simulink model "falseValue1"  (R2023a)
settings: Solver=VariableStepAuto  StartTime=0.0  StopTime=10.0  RelTol=1e-3
settings Model: Creator=Martin  LastModifiedBy=Martin

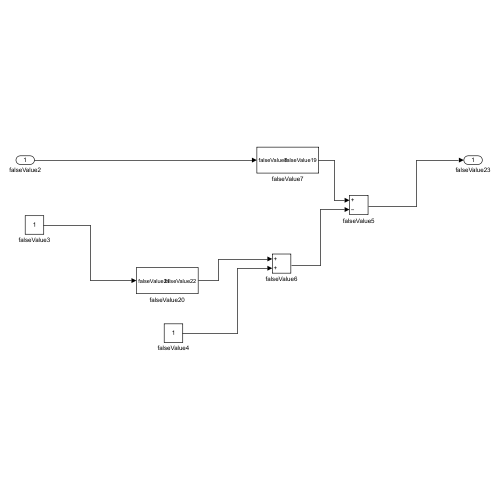
[thumbnail: Simulink's stored preview of the top-level diagram]
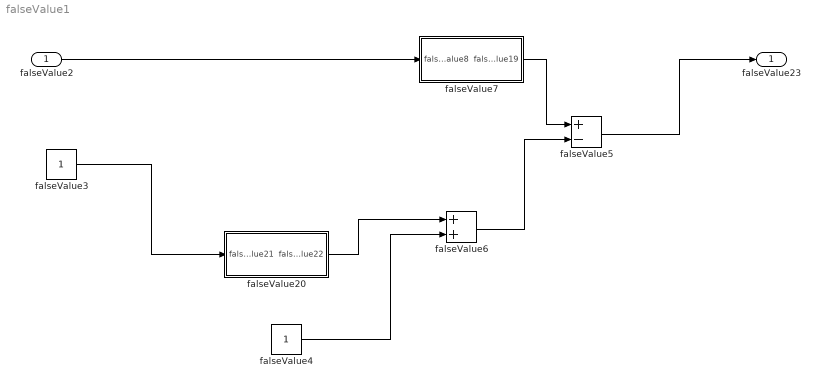
== system falseValue1 ==
  falseValue2 : Inport
  falseValue20 : Subsystem
  falseValue3 : Constant
  falseValue4 : Constant
  falseValue5 : Sum  Inputs=+-
  falseValue6 : Sum
  falseValue7 : Subsystem
  falseValue23 : Outport
  wires:
  falseValue2/1 -> falseValue7/1(falseValue8)
  falseValue5/1 -> falseValue23/1
  falseValue20/1(falseValue22) -> falseValue6/1
  falseValue4/1 -> falseValue6/2
  falseValue7/1(falseValue19) -> falseValue5/1
  falseValue6/1 -> falseValue5/2
  falseValue3/1 -> falseValue20/1(falseValue21)

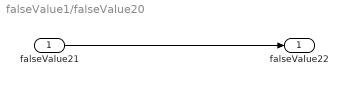
== system falseValue1/falseValue20 ==
  falseValue21 : Inport
  falseValue22 : Outport
  wires:
  falseValue21/1 -> falseValue22/1

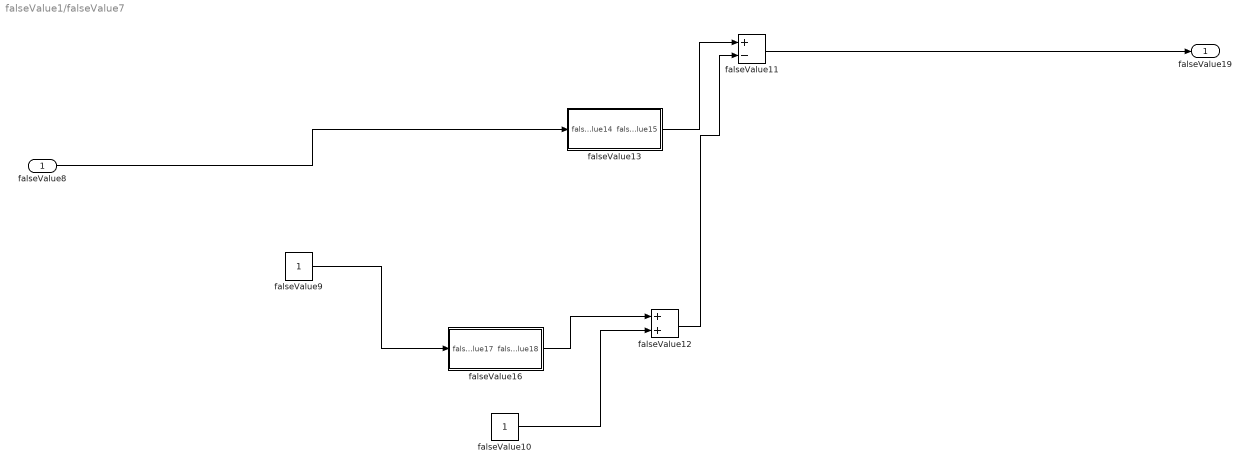
== system falseValue1/falseValue7 ==
  falseValue8 : Inport
  falseValue10 : Constant
  falseValue11 : Sum  Inputs=+-
  falseValue12 : Sum
  falseValue13 : Subsystem
  falseValue16 : Subsystem
  falseValue9 : Constant
  falseValue19 : Outport
  wires:
  falseValue9/1 -> falseValue16/1(falseValue17)
  falseValue12/1 -> falseValue11/2
  falseValue10/1 -> falseValue12/2
  falseValue16/1(falseValue18) -> falseValue12/1
  falseValue13/1(falseValue15) -> falseValue11/1
  falseValue8/1 -> falseValue13/1(falseValue14)
  falseValue11/1 -> falseValue19/1

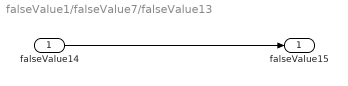
== system falseValue1/falseValue7/falseValue13 ==
  falseValue14 : Inport
  falseValue15 : Outport
  wires:
  falseValue14/1 -> falseValue15/1

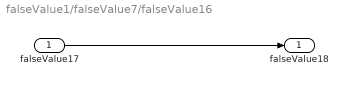
== system falseValue1/falseValue7/falseValue16 ==
  falseValue17 : Inport
  falseValue18 : Outport
  wires:
  falseValue17/1 -> falseValue18/1
